simulink model "Visualisation"  (R2022b)
settings: Solver=VariableStepAuto  StartTime=0.0  StopTime=10.0  RelTol=1e-3
settings Model: Creator=simon  LastModifiedBy=simon

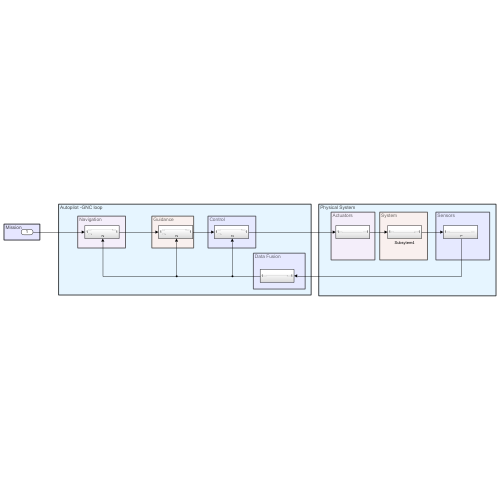
[thumbnail: Simulink's stored preview of the top-level diagram]
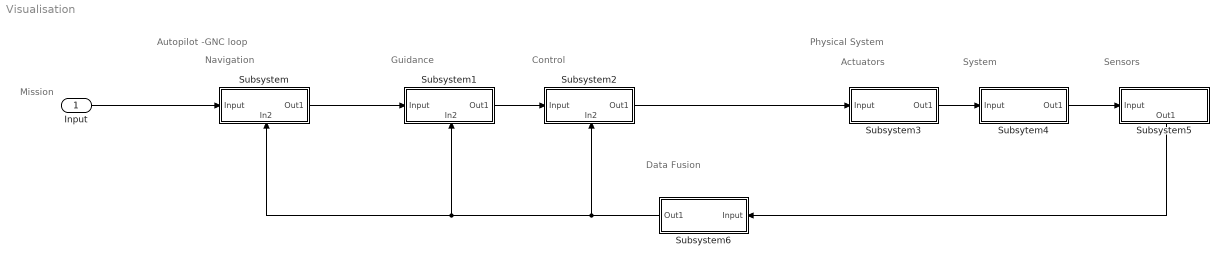
== system Visualisation ==
  note: Physical System
  note: Autopilot -GNC loop
  note: Navigation
  note: Mission
  note: Guidance
  note: Control
  note: Data Fusion
  note: Actuators
  note: System
  note: Sensors
  Input : Inport
  Subsystem : Subsystem
      settings: PortSchema="{\"entries\":[{\"content\":{\"sides\":[{\"content\":{\"connectorIds\":[\"In1\"]},\"type\":\"ConnectorPlacement.EquallySpacedRectSide\",\"uuid\":\"2eb23210-3dea-4b77-a9d4-7110bad0c58c\"},{\"content\":{\"connectorIds\":[\"Out1\"],\"side\":\"RIGHT\"},\"type\":\"ConnectorPlacement.EquallySpacedRectSide\",\"uuid\":\"94c709a1-e7e1-4346-819b-fd02519f91fd\"},{\"content\":{\"connectorIds\":[],\"side\":\"TOP\"},\"type\":\"ConnectorPlacement.EquallySpacedRectSide\",\"uuid\":\"53af2cc2-9550-447d-847d-ecbf9bed457e\"},{\"content\":{\"connectorIds\":[\"In2\"],\"side\":\"BOTTOM\"},\"type\":\"ConnectorPlacement.EquallySpacedRectSide\",\"uuid\":\"b16a108a-7c5f-4f66-a73b-13f2bc9d7ac4\"}]},\"type\":\"ConnectorPlacement.EquallySpacedConnector\",\"uuid\":\"16662f53-7def-47cf-8bdf-f2fc9af7dce9\"}],\"packageUris\":[\"http://schema.mathworks.com/mf0/Connector/R2020b\"],\"version\":\"1.0\"}"
  Subsystem1 : Subsystem
      settings: PortSchema="{\"entries\":[{\"content\":{\"sides\":[{\"content\":{\"connectorIds\":[\"In1\"]},\"type\":\"ConnectorPlacement.EquallySpacedRectSide\",\"uuid\":\"2eb23210-3dea-4b77-a9d4-7110bad0c58c\"},{\"content\":{\"connectorIds\":[\"Out1\"],\"side\":\"RIGHT\"},\"type\":\"ConnectorPlacement.EquallySpacedRectSide\",\"uuid\":\"94c709a1-e7e1-4346-819b-fd02519f91fd\"},{\"content\":{\"connectorIds\":[],\"side\":\"TOP\"},\"type\":\"ConnectorPlacement.EquallySpacedRectSide\",\"uuid\":\"53af2cc2-9550-447d-847d-ecbf9bed457e\"},{\"content\":{\"connectorIds\":[\"In2\"],\"side\":\"BOTTOM\"},\"type\":\"ConnectorPlacement.EquallySpacedRectSide\",\"uuid\":\"c0cb6d07-421f-4c5f-9ed6-902a152412e2\"}]},\"type\":\"ConnectorPlacement.EquallySpacedConnector\",\"uuid\":\"16662f53-7def-47cf-8bdf-f2fc9af7dce9\"}],\"packageUris\":[\"http://schema.mathworks.com/mf0/Connector/R2020b\"],\"version\":\"1.0\"}"
  Subsystem2 : Subsystem
      settings: PortSchema="{\"entries\":[{\"content\":{\"sides\":[{\"content\":{\"connectorIds\":[\"In1\"]},\"type\":\"ConnectorPlacement.EquallySpacedRectSide\",\"uuid\":\"2eb23210-3dea-4b77-a9d4-7110bad0c58c\"},{\"content\":{\"connectorIds\":[\"Out1\"],\"side\":\"RIGHT\"},\"type\":\"ConnectorPlacement.EquallySpacedRectSide\",\"uuid\":\"94c709a1-e7e1-4346-819b-fd02519f91fd\"},{\"content\":{\"connectorIds\":[],\"side\":\"TOP\"},\"type\":\"ConnectorPlacement.EquallySpacedRectSide\",\"uuid\":\"53af2cc2-9550-447d-847d-ecbf9bed457e\"},{\"content\":{\"connectorIds\":[\"In2\"],\"side\":\"BOTTOM\"},\"type\":\"ConnectorPlacement.EquallySpacedRectSide\",\"uuid\":\"c05d524f-d38c-4e64-bf10-135334aee553\"}]},\"type\":\"ConnectorPlacement.EquallySpacedConnector\",\"uuid\":\"16662f53-7def-47cf-8bdf-f2fc9af7dce9\"}],\"packageUris\":[\"http://schema.mathworks.com/mf0/Connector/R2020b\"],\"version\":\"1.0\"}"
  Subsystem3 : Subsystem
  Subsystem5 : Subsystem
      settings: PortSchema="{\"entries\":[{\"content\":{\"sides\":[{\"content\":{\"connectorIds\":[\"In1\"]},\"type\":\"ConnectorPlacement.EquallySpacedRectSide\",\"uuid\":\"2eb23210-3dea-4b77-a9d4-7110bad0c58c\"},{\"content\":{\"connectorIds\":[],\"side\":\"RIGHT\"},\"type\":\"ConnectorPlacement.EquallySpacedRectSide\",\"uuid\":\"94c709a1-e7e1-4346-819b-fd02519f91fd\"},{\"content\":{\"connectorIds\":[],\"side\":\"TOP\"},\"type\":\"ConnectorPlacement.EquallySpacedRectSide\",\"uuid\":\"53af2cc2-9550-447d-847d-ecbf9bed457e\"},{\"content\":{\"connectorIds\":[\"Out1\"],\"side\":\"BOTTOM\"},\"type\":\"ConnectorPlacement.EquallySpacedRectSide\",\"uuid\":\"b1df5d71-6836-4899-8e9d-10bba38a631d\"}]},\"type\":\"ConnectorPlacement.EquallySpacedConnector\",\"uuid\":\"16662f53-7def-47cf-8bdf-f2fc9af7dce9\"}],\"packageUris\":[\"http://schema.mathworks.com/mf0/Connector/R2020b\"],\"version\":\"1.0\"}"
  Subsystem6 : Subsystem
  Subsytem4 : Subsystem
  wires:
  Input/1 -> Subsystem/1(Input)
  Subsystem/1(Out1) -> Subsystem1/1(Input)
  Subsystem1/1(Out1) -> Subsystem2/1(Input)
  Subsystem2/1(Out1) -> Subsystem3/1(Input)
  Subsystem3/1(Out1) -> Subsytem4/1(Input)
  Subsytem4/1(Out1) -> Subsystem5/1(Input)
  Subsystem5/1(Out1) -> Subsystem6/1(Input)
  Subsystem6/1(Out1) -> Subsystem2/2(In2), Subsystem1/2(In2), Subsystem/2(In2)

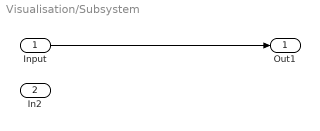
== system Visualisation/Subsystem ==
  Input : Inport
  In2 : Inport  Port=2
  Out1 : Outport
  wires:
  Input/1 -> Out1/1

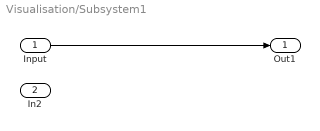
== system Visualisation/Subsystem1 ==
  Input : Inport
  In2 : Inport  Port=2
  Out1 : Outport
  wires:
  Input/1 -> Out1/1

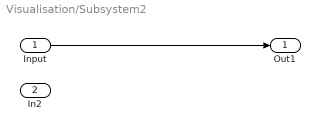
== system Visualisation/Subsystem2 ==
  Input : Inport
  In2 : Inport  Port=2
  Out1 : Outport
  wires:
  Input/1 -> Out1/1

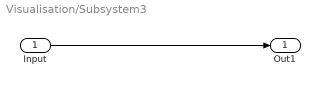
== system Visualisation/Subsystem3 ==
  Input : Inport
  Out1 : Outport
  wires:
  Input/1 -> Out1/1

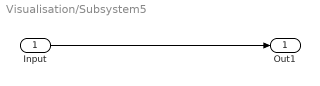
== system Visualisation/Subsystem5 ==
  Input : Inport
  Out1 : Outport
  wires:
  Input/1 -> Out1/1

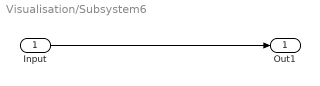
== system Visualisation/Subsystem6 ==
  Input : Inport
  Out1 : Outport
  wires:
  Input/1 -> Out1/1

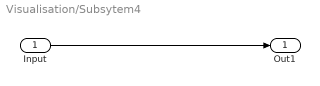
== system Visualisation/Subsytem4 ==
  Input : Inport
  Out1 : Outport
  wires:
  Input/1 -> Out1/1
